simulink model "Logic1"  (R2024a)
settings: Solver=FixedStepDiscrete  StartTime=0.0  StopTime=1  FixedStep=0.01  RelTol=1e-3
PostLoadFcn:
  | if any(exist('dsrtsu_mdlpostloadfcn', 'file') ~= 0), dsrtsu_mdlpostloadfcn('Execute', bdroot); end
InitFcn:
  | , if any(exist('rtifpga_mdlclblib', 'file') ~= 0), rtifpga_mdlclblib('Init', bdroot); end,
  | , if any(exist('dsmpb_private', 'file') ~= 0), dsmpb_private('dsmpb_mdlclblib', 'Init', bdroot); end,
libraries: simulink x1
PreSaveFcn:
  | , if any(exist('dsmpb_private', 'file') ~= 0), dsmpb_private('dsmpb_mdlclblib', 'PreSave', bdroot); end,
CloseFcn:
  | , if any(exist('dsmpb_private', 'file') ~= 0), dsmpb_private('dsmpb_mdlclblib', 'Close', bdroot); end,
settings Model: DSMPB_ID_DATA={}  DSRTSU_INTERNAL_RTIFPGA=210  Creator=sramakrishnan  LastModifiedBy=sramakrishnan
settings OptimizationCC: BlockReduction=off  ConditionallyExecuteInputs=off  OptimizeBlockIOStorage=off  BufferReuse=off
settings DebuggingCC: TasksWithSamePriorityMsg=none
settings HardwareCC: ProdBitPerPointer=32  ProdBitPerSizeT=32  ProdBitPerPtrDiffT=32  ProdLargestAtomicInteger=Integer  ProdWordSize=32  ProdLongLongMode=on  ProdHWDeviceType=Custom Processor->Custom
settings ModelReferenceCC: EnableParallelModelReferenceBuilds=on
settings RTWCC: Description=dSPACE Target DSRT - Generates SIC files for import by ConfigurationDesk and VEOS. Provides code generation for Simulink models imported in ConfigurationDesk.  SystemTargetFile=dsrt.tlc  GenCodeOnly=on  MakeCommand=make_dsrt  TemplateMakefile=dsrt_default_tmf  RTWVerbose=off
settings STFCustomTargetCC: ParMdlRefBuildCompliant=on  GRTInterface=off  UseToolchainInfoCompliant=off  SystemTargetFile=dsrt.tlc
settings GRTTargetCC: CompOptLevelCompliant=off  ConcurrentExecutionCompliant=off  CombineOutputUpdateFcns=off  MatFileLogging=off  CPPClassGenCompliant=off  UseToolchainInfoCompliant=off

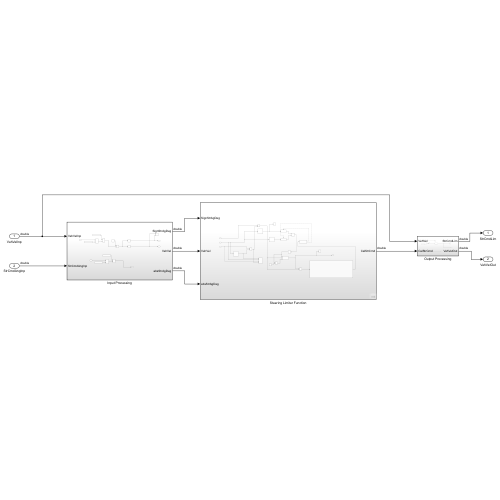
[thumbnail: Simulink's stored preview of the top-level diagram]
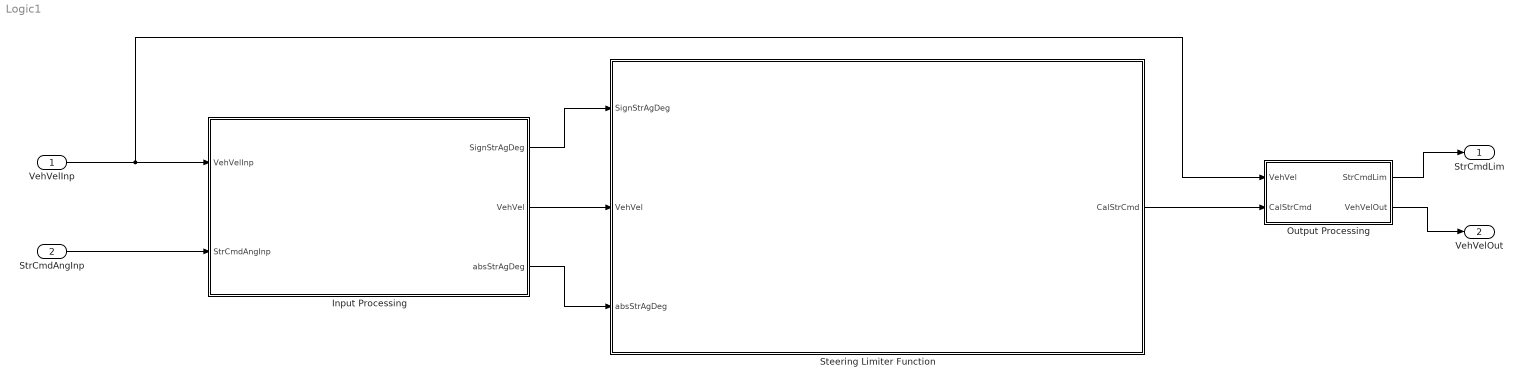
== system Logic1 ==
  VehVelInp : Inport
  StrCmdAngInp : Inport  Port=2
  Input Processing : Subsystem
  Output Processing : Subsystem
  Steering Limiter Function : Subsystem
  StrCmdLim : Outport
  VehVelOut : Outport  Port=2
  wires:
  Input Processing/1(SignStrAgDeg) -> Steering Limiter Function/1(SignStrAgDeg)
  Input Processing/2(VehVel) -> Steering Limiter Function/2(VehVel)
  Input Processing/3(absStrAgDeg) -> Steering Limiter Function/3(absStrAgDeg)
  Steering Limiter Function/1(CalStrCmd) -> Output Processing/2(CalStrCmd)
  VehVelInp/1 -> Output Processing/1(VehVel), Input Processing/1(VehVelInp)
  StrCmdAngInp/1 -> Input Processing/2(StrCmdAngInp)
  Output Processing/1(StrCmdLim) -> StrCmdLim/1
  Output Processing/2(VehVelOut) -> VehVelOut/1

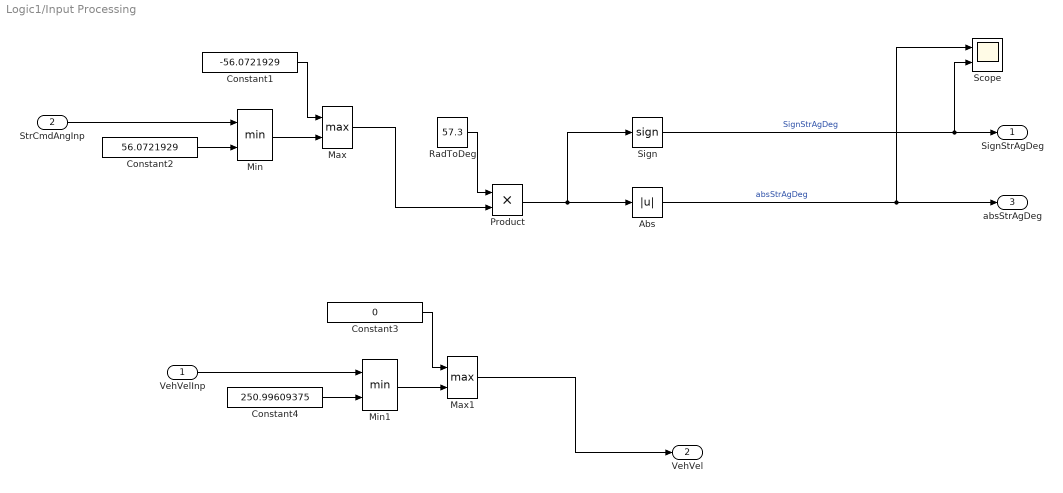
== system Logic1/Input Processing ==
  VehVelInp : Inport
  StrCmdAngInp : Inport  Port=2
  Abs : Abs  SaturateOnIntegerOverflow=off
  Constant1 : Constant  Value=-56.0721929
  Constant2 : Constant  Value=56.0721929
  Constant3 : Constant  Value=0
  Constant4 : Constant  Value=250.99609375
  Max : MinMax  Function=max  Inputs=2
  Max1 : MinMax  Function=max  Inputs=2
  Min : MinMax  Inputs=2
  Min1 : MinMax  Inputs=2
  Product : Product
  RadToDeg : Constant  Value=57.3
  Scope : Scope  NumInputPorts=2
  Sign : Signum
  SignStrAgDeg : Outport
  VehVel : Outport  Port=2
  absStrAgDeg : Outport  Port=3
  wires:
  Sign/1 -> Scope/2, SignStrAgDeg/1  "SignStrAgDeg"
  Product/1 -> Sign/1, Abs/1
  RadToDeg/1 -> Product/1
  Abs/1 -> Scope/1, absStrAgDeg/1  "absStrAgDeg"
  Constant2/1 -> Min/2
  StrCmdAngInp/1 -> Min/1
  Min/1 -> Max/2
  Constant1/1 -> Max/1
  Max/1 -> Product/2
  Min1/1 -> Max1/2
  Constant4/1 -> Min1/2
  Constant3/1 -> Max1/1
  Max1/1 -> VehVel/1
  VehVelInp/1 -> Min1/1

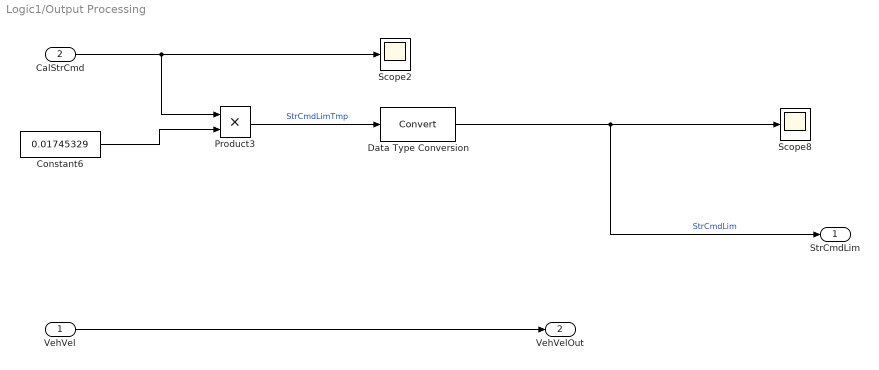
== system Logic1/Output Processing ==
  VehVel : Inport
  CalStrCmd : Inport  Port=2
  Constant6 : Constant  Value=0.01745329
  Data Type Conversion : DataTypeConversion  SaturateOnIntegerOverflow=off  RndMeth=Floor
  Product3 : Product
  Scope2 : Scope
  Scope8 : Scope
  StrCmdLim : Outport
  VehVelOut : Outport  Port=2
  wires:
  Product3/1 -> Data Type Conversion/1  "StrCmdLimTmp"
  Constant6/1 -> Product3/2
  CalStrCmd/1 -> Product3/1, Scope2/1
  VehVel/1 -> VehVelOut/1
  Data Type Conversion/1 -> StrCmdLim/1, Scope8/1  "StrCmdLim"

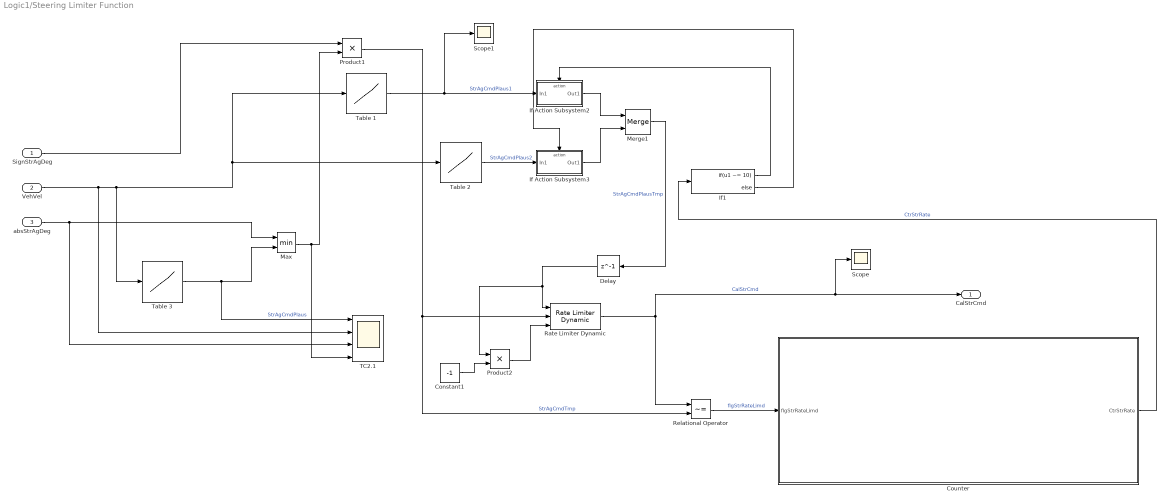
== system Logic1/Steering Limiter Function ==
  SignStrAgDeg : Inport
  VehVel : Inport  Port=2
  absStrAgDeg : Inport  Port=3
  Constant1 : Constant  Value=-1
  Counter : Subsystem
  Delay : Delay  DelayLength=1
  If Action Subsystem2 : Subsystem  TreatAsAtomicUnit=on
  If Action Subsystem3 : Subsystem  TreatAsAtomicUnit=on
  If1 : If  IfExpression=u1 ~= 10
  Max : MinMax  Inputs=2
  Merge1 : Merge
  Product1 : Product
  Product2 : Product
  Rate Limiter Dynamic : simulink/Discontinuities/Rate Limiter Dynamic
  Relational Operator : RelationalOperator  Operator=~=  OutDataTypeStr=boolean  RndMeth=Simplest  InputSameDT=off
  Scope : Scope
  Scope1 : Scope
  TC2.1 : Scope  NumInputPorts=4
  Table 1 : Lookup_n-D  NumberOfTableDimensions=1  BreakpointsForDimension1=[0;8.04672;16.09344;24.14016;32.18688;40.2336;56.32704;72.42048;88.51392;104.6074]  Table=[479.9834;479.9834;462.5181;426.2757;312.5545;267.5176;244.988;214.9901;190.0149;155.0244]  ExtrapMethod=Clip  UseLastTableValue=on  InternalRulePriority=Speed  RndMeth=Simplest
  Table 2 : Lookup_n-D  NumberOfTableDimensions=1  BreakpointsForDimension1=[0;8.04672;16.09344;24.14016;32.18688;40.2336;56.32704;72.42048;88.51392;104.6074]  Table=[299.4082;275.0638;238.546;214.2657;202.2014;178.0706;58.8714;11.773;8.2405;5.8876]  ExtrapMethod=Clip  UseLastTableValue=on  InternalRulePriority=Speed  RndMeth=Simplest
  Table 3 : Lookup_n-D  NumberOfTableDimensions=1  BreakpointsForDimension1=[0;10.00008;20.00016;29.99988;39.99996;50;60.00012;69.99984;79.99992;90]  Table=[943.4003;943.4003;776.0209;378.4347;221.4865;148.229;121.0109;100.0285;85.4008;74.9696]  ExtrapMethod=Clip  UseLastTableValue=on  InternalRulePriority=Speed  RndMeth=Simplest
  CalStrCmd : Outport
  wires:
  If1/2 -> If Action Subsystem3/Action
  If Action Subsystem2/1(Out1) -> Merge1/1
  Product1/1 -> Relational Operator/2, Rate Limiter Dynamic/2  "StrAgCmdTmp"
  VehVel/1 -> TC2.1/2, Table 1/1, Table 2/1, Table 3/1
  Product2/1 -> Rate Limiter Dynamic/3
  Rate Limiter Dynamic/1 -> Relational Operator/1, Scope/1, CalStrCmd/1  "CalStrCmd"
  Table 3/1 -> TC2.1/1, Max/2  "StrAgCmdPlaus"
  If Action Subsystem3/1(Out1) -> Merge1/2
  Constant1/1 -> Product2/2
  If1/1 -> If Action Subsystem2/Action
  Merge1/1 -> Delay/1  "StrAgCmdPlausTmp"
  Max/1 -> TC2.1/4, Product1/2
  absStrAgDeg/1 -> TC2.1/3, Max/1
  SignStrAgDeg/1 -> Product1/1
  Relational Operator/1 -> Counter/1(flgStrRateLimd)  "flgStrRateLimd"
  Counter/1(CtrStrRate) -> If1/1  "CtrStrRate"
  Table 1/1 -> Scope1/1, If Action Subsystem2/1(In1)  "StrAgCmdPlaus1"
  Table 2/1 -> If Action Subsystem3/1(In1)  "StrAgCmdPlaus2"
  Delay/1 -> Rate Limiter Dynamic/1, Product2/1

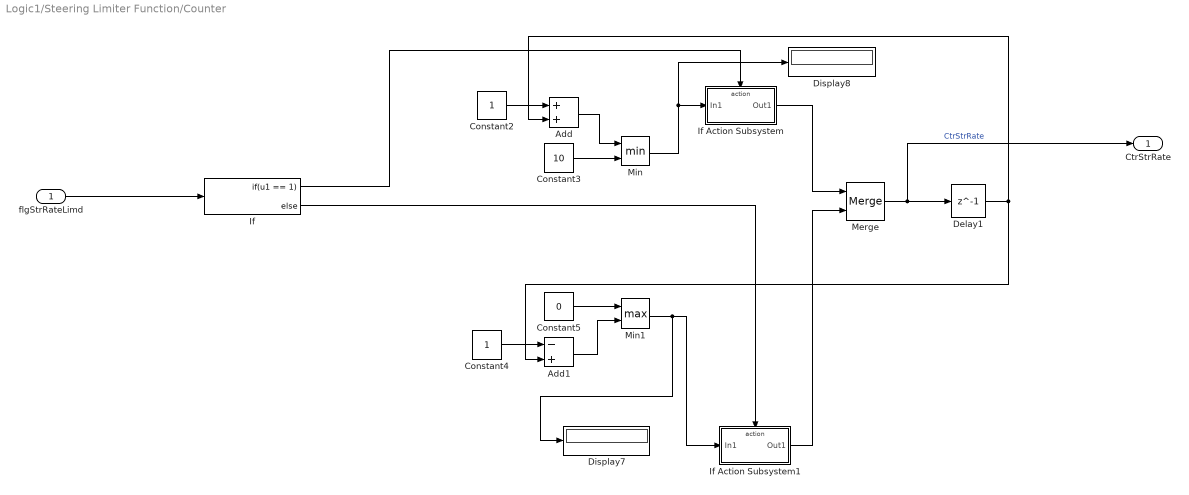
== system Logic1/Steering Limiter Function/Counter ==
  flgStrRateLimd : Inport
  Add : Sum
  Add1 : Sum  Inputs=-+
  Constant2 : Constant
  Constant3 : Constant  Value=10
  Constant4 : Constant
  Constant5 : Constant  Value=0
  Delay1 : Delay  DelayLength=1
  Display7 : Display
  Display8 : Display
  If : If  IfExpression=u1 == 1
  If Action Subsystem : Subsystem  TreatAsAtomicUnit=on
  If Action Subsystem1 : Subsystem  TreatAsAtomicUnit=on
  Merge : Merge
  Min : MinMax  Inputs=2
  Min1 : MinMax  Function=max  Inputs=2
  CtrStrRate : Outport
  wires:
  Constant3/1 -> Min/2
  Add/1 -> Min/1
  If/1 -> If Action Subsystem/Action
  Constant2/1 -> Add/1
  Constant5/1 -> Min1/1
  Constant4/1 -> Add1/1
  Merge/1 -> CtrStrRate/1, Delay1/1  "CtrStrRate"
  Min/1 -> Display8/1, If Action Subsystem/1(In1)
  Add1/1 -> Min1/2
  If Action Subsystem1/1(Out1) -> Merge/2
  Delay1/1 -> Add1/2, Add/2
  Min1/1 -> Display7/1, If Action Subsystem1/1(In1)
  If Action Subsystem/1(Out1) -> Merge/1
  If/2 -> If Action Subsystem1/Action
  flgStrRateLimd/1 -> If/1

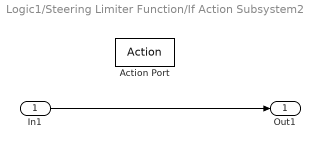
== system Logic1/Steering Limiter Function/If Action Subsystem2 ==
  In1 : Inport
  Action Port : ActionPort  ActionPortLabel=if(u1 ~= 10)
  Out1 : Outport
  wires:
  In1/1 -> Out1/1

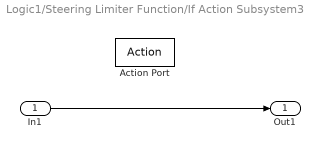
== system Logic1/Steering Limiter Function/If Action Subsystem3 ==
  In1 : Inport
  Action Port : ActionPort  ActionPortLabel=else
  Out1 : Outport
  wires:
  In1/1 -> Out1/1

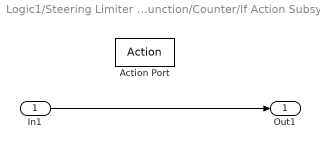
== system Logic1/Steering Limiter Function/Counter/If Action Subsystem ==
  In1 : Inport
  Action Port : ActionPort  ActionPortLabel=if(u1 == 1)
  Out1 : Outport
  wires:
  In1/1 -> Out1/1

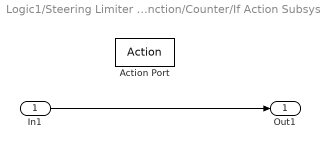
== system Logic1/Steering Limiter Function/Counter/If Action Subsystem1 ==
  In1 : Inport
  Action Port : ActionPort  ActionPortLabel=else
  Out1 : Outport
  wires:
  In1/1 -> Out1/1
